simulink model "aerobrakesim"  (R2024a)
settings: Solver=VariableStepAuto  StartTime=0.0  StopTime=P.tv(end)  RelTol=1e-3
values from neighbouring files (symbols this model uses):
  forces = uu(k)    [aerobrakesim_kin_dyn.m]    (also in aerobrakesim_sensors.m)
  P = []    [init_aerobrakesim_params.m]    (also in load_aerobrakesim.m = init_aerobrakesim_params)
undefined symbols (not defined in the file or in its folder): aerobrakesim_control, aerobrakesim_estimates, aerobrakesim_forces_moments, aerobrakesim_kin_dyn, aerobrakesim_logging, aerobrakesim_sensors, aerobrakesim_trajectory_control
settings Model: Creator=Dimit  LastModifiedBy=Dimit

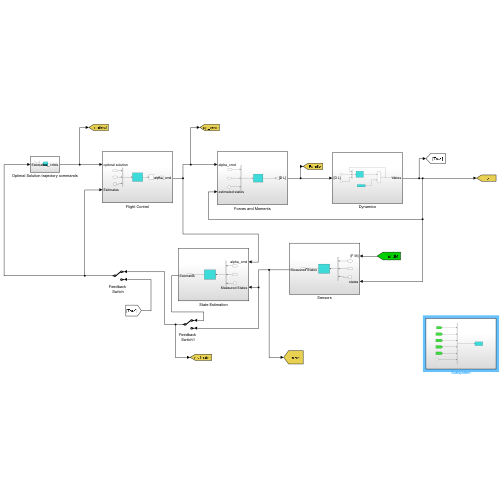
[thumbnail: Simulink's stored preview of the top-level diagram]
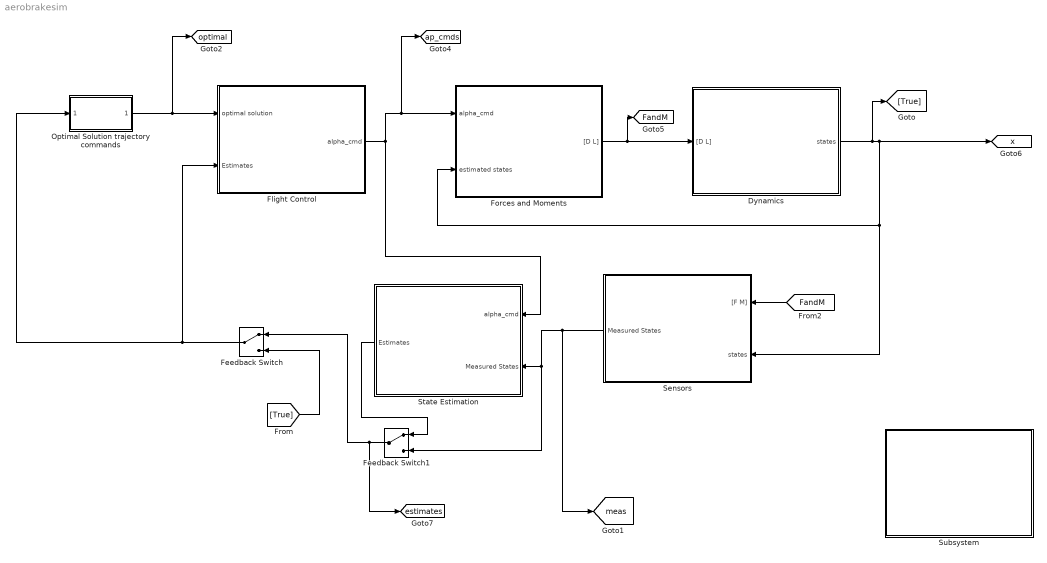
== system aerobrakesim ==
  Dynamics : Subsystem
  Feedback Switch : ManualSwitch
  Feedback Switch1 : ManualSwitch
  Flight Control : Subsystem
  Forces and Moments : Subsystem
  Optimal Solution trajectory commands : Subsystem
  Sensors : Subsystem
  State Estimation : Subsystem
  Subsystem : Subsystem
  tag scope: FandM=global, ap_cmds=global, estimates=global, meas=global, optimal=global, x=global
  wires:
  Forces and Moments/1("[D L]") -> [FandM], Dynamics/1("[D L]")
  [FandM] -> Sensors/1("[F M]")
  [True] -> Feedback Switch/2
  Feedback Switch/1 -> Flight Control/2(Estimates), Optimal Solution trajectory commands/1(Estimates)
  Sensors/1(Measured States) -> [meas], Feedback Switch1/2, State Estimation/2(Measured States)
  State Estimation/1(Estimates) -> Feedback Switch1/1
  Feedback Switch1/1 -> [estimates], Feedback Switch/1
  Dynamics/1(states) -> [True], [x], Forces and Moments/2(estimated states), Sensors/2(states)
  Flight Control/1(alpha_cmd) -> State Estimation/1(alpha_cmd), [ap_cmds], Forces and Moments/1(alpha_cmd)
  Optimal Solution trajectory commands/1(traj_cmds) -> [optimal], Flight Control/1(optimal solution)

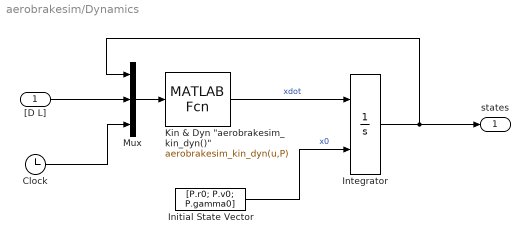
== system aerobrakesim/Dynamics ==
  "[D L]" : Inport
  Clock : Clock
  Initial State Vector : Constant  Value=[P.r0; P.v0; P.gamma0]
  Integrator : Integrator  InitialConditionSource=external
  "Kin & Dyn \"aerobrakesim_kin_dyn()\"" : MATLABFcn  MATLABFcn=aerobrakesim_kin_dyn(u,P)  OutputDimensions="3    % # of states"
  Mux : Mux  Inputs=3
  states : Outport  VectorParamsAs1DForOutWhenUnconnected=off
  wires:
  "Kin & Dyn \"aerobrakesim_kin_dyn()\""/1 -> Integrator/1  "xdot"
  Integrator/1 -> Mux/1, states/1
  Initial State Vector/1 -> Integrator/2  "x0"
  Mux/1 -> "Kin & Dyn \"aerobrakesim_kin_dyn()\""/1
  "[D L]"/1 -> Mux/2
  Clock/1 -> Mux/3

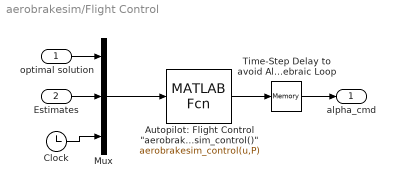
== system aerobrakesim/Flight Control ==
  optimal solution : Inport
  Estimates : Inport  Port=2
  "Autopilot: Flight Control \"aerobrakesim_control()\"" : MATLABFcn  MATLABFcn=aerobrakesim_control(u,P)  OutputDimensions=1  SampleTime="P.Ts     % Autopilot at 100Hz"
  Clock : Clock
  Mux : Mux  Inputs=3
  Time-Step Delay to avoid Algebraic Loop : Memory  InitialCondition=[P.uv(1)]'
  alpha_cmd : Outport
  wires:
  Mux/1 -> "Autopilot: Flight Control \"aerobrakesim_control()\""/1
  optimal solution/1 -> Mux/1
  Estimates/1 -> Mux/2
  Clock/1 -> Mux/3
  "Autopilot: Flight Control \"aerobrakesim_control()\""/1 -> Time-Step Delay to avoid Algebraic Loop/1
  Time-Step Delay to avoid Algebraic Loop/1 -> alpha_cmd/1

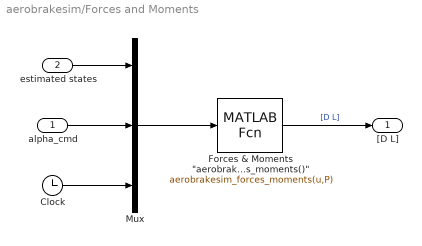
== system aerobrakesim/Forces and Moments ==
  alpha_cmd : Inport
  estimated states : Inport  Port=2
  Clock : Clock
  "Forces & Moments \"aerobrakesim_forces_moments()\"" : MATLABFcn  MATLABFcn=aerobrakesim_forces_moments(u,P)  OutputDimensions=2 % (2 forces)
  Mux : Mux  Inputs=3
  "[D L]" : Outport
  wires:
  "Forces & Moments \"aerobrakesim_forces_moments()\""/1 -> "[D L]"/1  "[D L]"
  Mux/1 -> "Forces & Moments \"aerobrakesim_forces_moments()\""/1
  alpha_cmd/1 -> Mux/2
  estimated states/1 -> Mux/1
  Clock/1 -> Mux/3

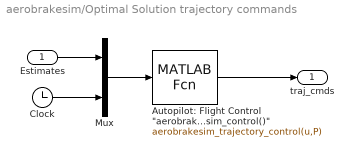
== system aerobrakesim/Optimal Solution trajectory commands ==
  Estimates : Inport
  "Autopilot: Flight Control \"aerobrakesim_control()\"" : MATLABFcn  MATLABFcn=aerobrakesim_trajectory_control(u,P)  OutputDimensions=4  SampleTime="P.Ts     % Autopilot at 100Hz"
  Clock : Clock
  Mux : Mux  Inputs=2
  traj_cmds : Outport
  wires:
  "Autopilot: Flight Control \"aerobrakesim_control()\""/1 -> traj_cmds/1
  Estimates/1 -> Mux/1
  Mux/1 -> "Autopilot: Flight Control \"aerobrakesim_control()\""/1
  Clock/1 -> Mux/2

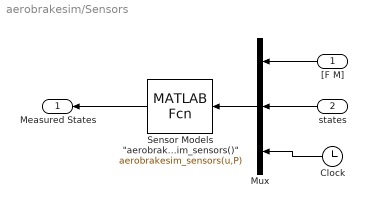
== system aerobrakesim/Sensors ==
  "[F M]" : Inport
  states : Inport  Port=2
  Clock : Clock
  Mux : Mux  Inputs=3
  "Sensor Models \"aerobrakesim_sensors()\"" : MATLABFcn  MATLABFcn=aerobrakesim_sensors(u,P)  OutputDimensions=3  SampleTime=P.Ts
  Measured States : Outport
  wires:
  Mux/1 -> "Sensor Models \"aerobrakesim_sensors()\""/1
  "[F M]"/1 -> Mux/1
  states/1 -> Mux/2
  "Sensor Models \"aerobrakesim_sensors()\""/1 -> Measured States/1
  Clock/1 -> Mux/3

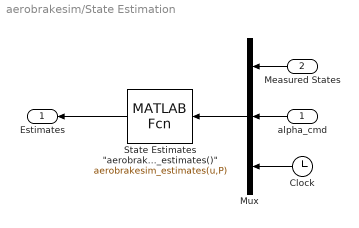
== system aerobrakesim/State Estimation ==
  alpha_cmd : Inport
  Measured States : Inport  Port=2
  Clock : Clock
  Mux : Mux  Inputs=3
  "State Estimates \"aerobrakesim_estimates()\"" : MATLABFcn  MATLABFcn=aerobrakesim_estimates(u,P)  OutputDimensions=3  SampleTime="P.Ts   % Autopilot at 100 Hz"
  Estimates : Outport
  wires:
  "State Estimates \"aerobrakesim_estimates()\""/1 -> Estimates/1
  Mux/1 -> "State Estimates \"aerobrakesim_estimates()\""/1
  Clock/1 -> Mux/3
  Measured States/1 -> Mux/1
  alpha_cmd/1 -> Mux/2

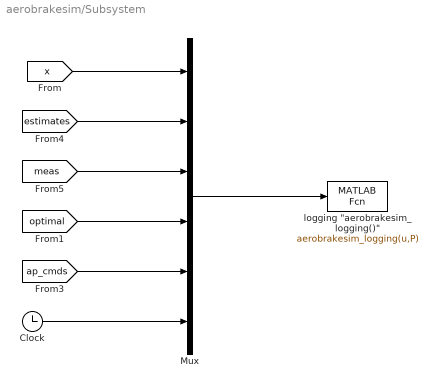
== system aerobrakesim/Subsystem ==
  Clock : Clock
  Mux : Mux  Inputs=6
  "logging \"aerobrakesim_logging()\"" : MATLABFcn  MATLABFcn=aerobrakesim_logging(u,P)  OutputDimensions=0  SampleTime=P.Tlog
  wires:
  [x] -> Mux/1
  [estimates] -> Mux/2
  [meas] -> Mux/3
  [ap_cmds] -> Mux/5
  Clock/1 -> Mux/6
  [optimal] -> Mux/4
  Mux/1 -> "logging \"aerobrakesim_logging()\""/1
